simulink model "ejercicio5"  (R2022b)
settings: Solver=VariableStepAuto  StartTime=0.0  StopTime=10.0  RelTol=1e-3
settings Model: Creator=Fran  LastModifiedBy=Fran

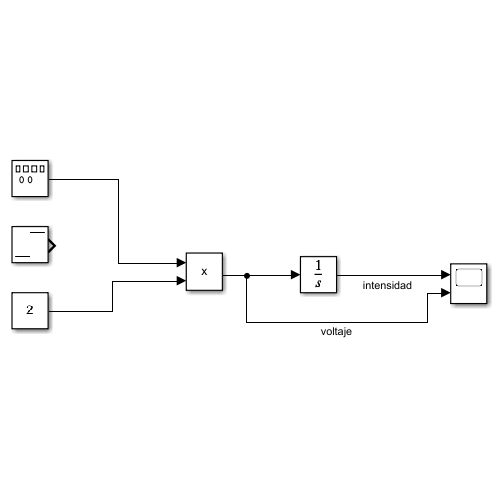
[thumbnail: Simulink's stored preview of the top-level diagram]
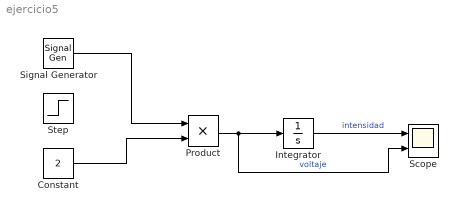
== system ejercicio5 ==
  Constant : Constant  Value=2
  Integrator : Integrator
  Product : Product
  Scope : Scope  NumInputPorts=2
  Signal Generator : SignalGenerator  Frequency=0.2
  Step : Step  Time=0  SampleTime=0
  wires:
  Constant/1 -> Product/2
  Integrator/1 -> Scope/1  "intensidad"
  Product/1 -> Scope/2, Integrator/1  "voltaje"
  Signal Generator/1 -> Product/1
